simulink model "AAI"  (R2022a)
settings: Solver=FixedStepAuto  StartTime=0.0  StopTime=10.0  FixedStep=1e-3  RelTol=1e-3  EnableMultiTasking=on
undefined symbols (not defined in the file): D0, D10, D11, D12, D13, D2, D4, D5, D6, D7, D8, D9, PTA0, PTA2, PTB23, PTB9, PTC16, PTC2, PTC3, PTC4, PTD0, PTD1, PTD2, PTD3
libraries: frdmk64flib x14
settings Model: ExtModeTrigDuration=5  Creator=jacqu  LastModifiedBy=jacqu
settings OptimizationCC: EnhancedBackFolding=on  PassReuseOutputArgsAs=Individual arguments  ZeroExternalMemoryAtStartup=off  ZeroInternalMemoryAtStartup=off  MaxStackSize=64  OptimizeBlockOrder=speed  DifferentSizesBufferReuse=on  OptimizationCustomize=off  EfficientTunableParamExpr=on
settings DebuggingCC: ParameterTunabilityLossMsg=error
settings HardwareCC: ProdBitPerPointer=32  ProdBitPerSizeT=32  ProdBitPerPtrDiffT=32  ProdLargestAtomicInteger=Long  ProdLargestAtomicFloat=Double  ProdWordSize=32  ProdHWDeviceType=ARM Compatible->ARM Cortex
settings SFSimCC: MATLABDynamicMemAlloc=off
settings RTWCC: SystemTargetFile=ert.tlc  HardwareBoard=NXP FRDM-K64F  TLCOptions="-aInlineSetEventsForThisBaseRateFcn=TLC_FALSE -aSuppressMultiTaskScheduler=TLC_FALSE  -aRateBasedStepFcn=0"  TemplateMakefile=ert_default_tmf  Toolchain=GNU Tools for ARM Embedded Processors
settings CodeAppCC: ForceParamTrailComments=on  IgnoreCustomStorageClasses=off  OperatorAnnotations=on  SimulinkDataObjDesc=on  SFDataObjDesc=on  InsertBlockDesc=on
settings ERTTargetCC: ExtModeTransport=4  ExtModeMexFile=sendToCommService

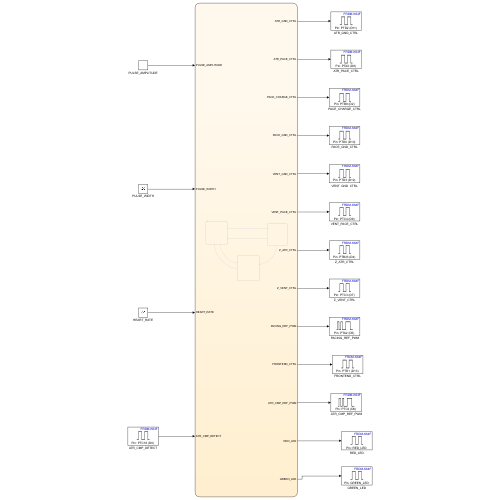
[thumbnail: Simulink's stored preview of the top-level diagram]
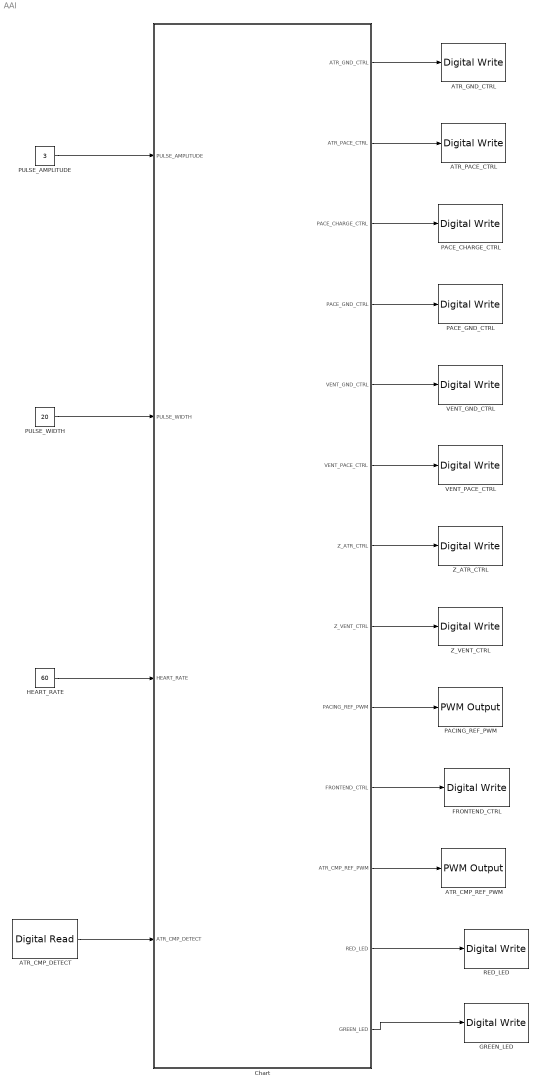
== system AAI ==
  " ATR_CMP_REF_PWM" : frdmk64flib/PWM Output  Whichpin=PTC2 (D6)  InitialFrequency=2000  InitialDutyCycle=0
  " PACING_REF_PWM" : frdmk64flib/PWM Output  Whichpin=PTA2 (D5)  InitialFrequency=2000  InitialDutyCycle=0
  ATR_CMP_DETECT : frdmk64flib/Digital Read  Whichpin=PTC16 (D0)  SampleTime=-1
  ATR_GND_CTRL : frdmk64flib/Digital Write  Whichpin=PTD2 (D11)
  ATR_PACE_CTRL : frdmk64flib/Digital Write  Whichpin=PTA0 (D8)
  Chart : Stateflow chart  TreatAsAtomicUnit=on
  FRONTEND_CTRL : frdmk64flib/Digital Write  Whichpin=PTD1 (D13)
  GREEN_LED : frdmk64flib/Digital Write  Whichpin=GREEN_LED
  HEART_RATE : Constant  Value=60
  PACE_CHARGE_CTRL : frdmk64flib/Digital Write  Whichpin=PTB9 (D2)
  PACE_GND_CTRL : frdmk64flib/Digital Write  Whichpin=PTD0 (D10)
  PULSE_AMPLITUDE : Constant  Value=3
  PULSE_WIDTH : Constant  Value=20
  RED_LED : frdmk64flib/Digital Write  Whichpin=RED_LED
  VENT_GND_CTRL : frdmk64flib/Digital Write  Whichpin=PTD3 (D12)
  VENT_PACE_CTRL : frdmk64flib/Digital Write  Whichpin=PTC4 (D9)
  Z_ATR_CTRL : frdmk64flib/Digital Write  Whichpin=PTB23 (D4)
  Z_VENT_CTRL : frdmk64flib/Digital Write  Whichpin=PTC3 (D7)
  wires:
  Chart/1(ATR_GND_CTRL) -> ATR_GND_CTRL/1
  Chart/2(ATR_PACE_CTRL) -> ATR_PACE_CTRL/1
  Chart/3(PACE_CHARGE_CTRL) -> PACE_CHARGE_CTRL/1
  Chart/4(PACE_GND_CTRL) -> PACE_GND_CTRL/1
  Chart/5(VENT_GND_CTRL) -> VENT_GND_CTRL/1
  Chart/6(VENT_PACE_CTRL) -> VENT_PACE_CTRL/1
  Chart/7(Z_ATR_CTRL) -> Z_ATR_CTRL/1
  Chart/8(Z_VENT_CTRL) -> Z_VENT_CTRL/1
  Chart/9(PACING_REF_PWM) -> " PACING_REF_PWM"/1
  Chart/10(FRONTEND_CTRL) -> FRONTEND_CTRL/1
  Chart/12(RED_LED) -> RED_LED/1
  Chart/13(GREEN_LED) -> GREEN_LED/1
  HEART_RATE/1 -> Chart/3(HEART_RATE)
  PULSE_WIDTH/1 -> Chart/2(PULSE_WIDTH)
  PULSE_AMPLITUDE/1 -> Chart/1(PULSE_AMPLITUDE)
  ATR_CMP_DETECT/1 -> Chart/4(ATR_CMP_DETECT)
  Chart/11(ATR_CMP_REF_PWM) -> " ATR_CMP_REF_PWM"/1

== stateflow chart AAI/Chart ==
  state PACE_OFF
    entry:
    ATR_PACE_CTRL = 0
    VENT_PACE_CTRL = 0
    PACING_REF_PWM = 20*PULSE_AMPLITUDE
    PACE_CHARGE_CTRL = 1
    PACE_GND_CTRL = 1
    VENT_PACE_CTRL = 0
    Z_ATR_CTRL = 0
    Z_VENT_CTRL = 0
    ATR_PACE_CTRL = 0
    ATR_GND_CTRL = 1
    VENT_GND_CTRL = 0
    FRONTEND_CTRL = 1
    ATR_CMP_REF_PWM = 20*PULSE_AMPLITUDE
    % light indicators
    RED_LED = 0
    GREEN_LED = 0
  state PACE_ON
    entry:
    PACE_CHARGE_CTRL = 0
    PACE_GND_CTRL = 1
    ATR_PACE_CTRL = 1
    ATR_GND_CTRL = 0
    Z_ATR_CTRL = 0
    Z_VENT_CTRL = 0
    VENT_GND_CTRL = 0
    VENT_PACE_CTRL = 0
    % light indicator
    RED_LED = 1
  state REFRACTORY
    entry:
    FRONTEND_CTRL = 0
    ATR_PACE_CTRL = 0
    ATR_GND_CTRL = 1
    PACING_REF_PWM = 20*PULSE_AMPLITUDE
    PACE_CHARGE_CTRL = 0
    PACE_GND_CTRL = 1
    % light indicator
    GREEN_LED = 1
  (default) -> PACE_OFF
  PACE_OFF -> PACE_ON [order 1] : [(ATR_CMP_DETECT == 0) & after((60000/HEART_RATE)-PULSE_WIDTH,msec)]
  PACE_ON -> PACE_OFF [order 2] : [after(PULSE_WIDTH, msec)]
  REFRACTORY -> PACE_OFF
  PACE_OFF -> REFRACTORY [order 2] : [ATR_CMP_DETECT == 1]
  PACE_ON -> REFRACTORY [order 1] : [ATR_CMP_DETECT == 1]
  data: ATR_GND_CTRL output; ATR_PACE_CTRL output; PACE_CHARGE_CTRL output; PACE_GND_CTRL output; VENT_GND_CTRL output; VENT_PACE_CTRL output; Z_ATR_CTRL output; Z_VENT_CTRL output; PULSE_AMPLITUDE input; PACING_REF_PWM output; FRONTEND_CTRL output; ATR_CMP_REF_PWM output; RED_LED output; PULSE_WIDTH input; HEART_RATE input; ATR_CMP_DETECT input; GREEN_LED output
